simulink model "sim_controller_from_ground"  (R2024b)
settings: Solver=ode1be  StartTime=t_0  StopTime=100  FixedStep=dt  RelTol=1e-8
undefined symbols (not defined in the file or in its folder): controller_rate
libraries: simulink x1
settings Model: Creator=yevge  LastModifiedBy=Aiden Gaydos
settings DebuggingCC: AlgebraicLoopMsg=error  CheckMatrixSingularityMsg=error

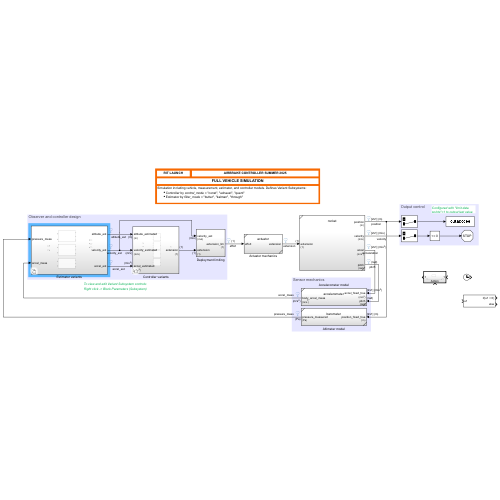
[thumbnail: Simulink's stored preview of the top-level diagram]
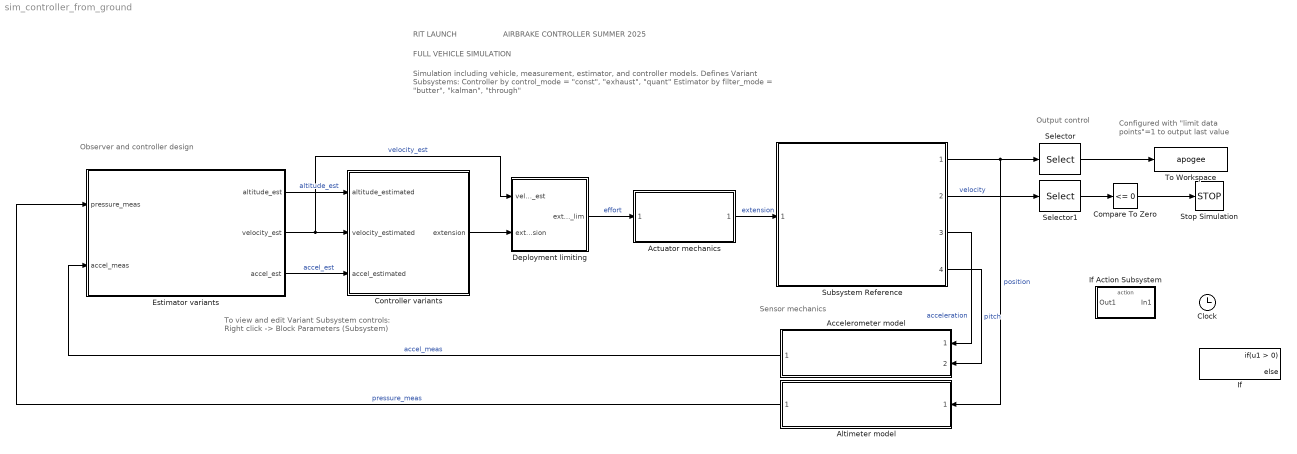
== system sim_controller_from_ground ==
  note: Output control
  note: Configured with "limit data points"=1 to output last value
  note: Sensor mechanics
  note: Observer and controller design
  note: AIRBRAKE CONTROLLER SUMMER 2025
  note: Simulation including vehicle, measurement, estimator, and controller models. Defines Variant Subsystems:
      | Controller by control_mode = "const", "exhaust", "quant"
      | Estimator by filter_mode = "butter", "kalman", "through"
  note: RIT LAUNCH
  note: FULL VEHICLE SIMULATION
  note: To view and edit Variant Subsystem controls:
      | Right click -> Block Parameters (Subsystem)
  Accelerometer model : Subsystem  ReferencedSubsystem=accelerometer
  Actuator mechanics : Subsystem  ReferencedSubsystem=actuator
  Altimeter model : Subsystem  ReferencedSubsystem=barometer
  Clock : Clock
  Compare To Zero : simulink/Logic and Bit Operations/Compare To Zero  relop=<=  OutDataTypeStr=boolean
  Controller variants : Subsystem  Variant=on  VariantControl=Subsystem  AllowZeroVariantControls=on
  Deployment limiting : Subsystem
  Estimator variants : Subsystem  Variant=on  VariantControl=Signal processing  AllowZeroVariantControls=on
  If : If
  If Action Subsystem : Subsystem  TreatAsAtomicUnit=on
  Selector : Selector  InputPortWidth=2  IndexOptions=Index vector (dialog)  Indices=2  OutputSizes=1
  Selector1 : Selector  InputPortWidth=2  IndexOptions=Index vector (dialog)  Indices=2  OutputSizes=1
  Stop Simulation : Stop
  Subsystem Reference : Subsystem  ReferencedSubsystem=rocket
  To Workspace : ToWorkspace  VariableName=apogee  SampleTime=-1
      settings: MaxDataPoints=1
  wires:
  Subsystem Reference/3 -> Accelerometer model/1  "acceleration"
  Subsystem Reference/4 -> Accelerometer model/2  "pitch"
  Subsystem Reference/1 -> Selector/1, Altimeter model/1  "position"
  Selector1/1 -> Compare To Zero/1
  Compare To Zero/1 -> Stop Simulation/1
  Selector/1 -> To Workspace/1
  Subsystem Reference/2 -> Selector1/1  "velocity"
  Controller variants/1(extension) -> Deployment limiting/2(extension)
  Deployment limiting/1(extension_lim) -> Actuator mechanics/1  "effort"
  Actuator mechanics/1 -> Subsystem Reference/1  "extension"
  Accelerometer model/1 -> Estimator variants/2(accel_meas)  "accel_meas"
  Estimator variants/1(altitude_est) -> Controller variants/1(altitude_estimated)  "altitude_est"
  Estimator variants/2(velocity_est) -> Controller variants/2(velocity_estimated), Deployment limiting/1(velocity_est)  "velocity_est"
  Estimator variants/3(accel_est) -> Controller variants/3(accel_estimated)  "accel_est"
  Altimeter model/1 -> Estimator variants/1(pressure_meas)  "pressure_meas"

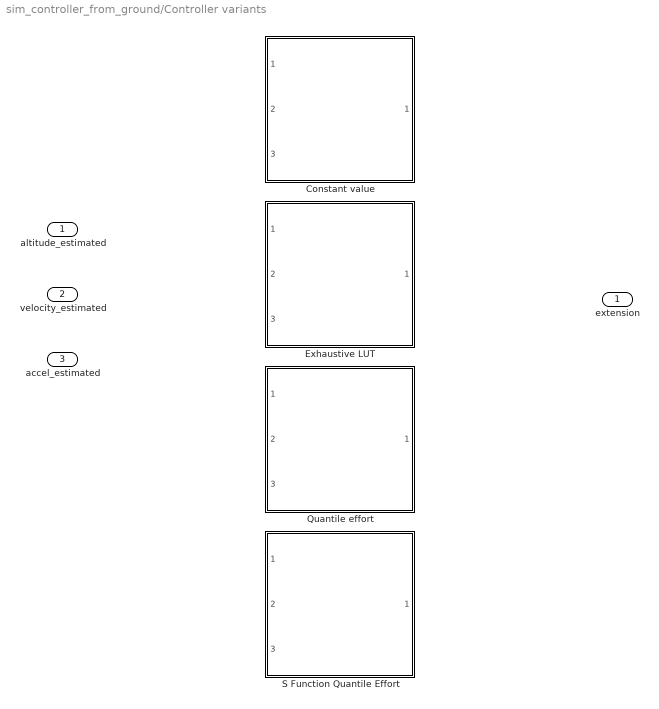
== system sim_controller_from_ground/Controller variants ==
  altitude_estimated : Inport  Unit=m  PortDimensions=1  SampleTime=1/controller_rate
  velocity_estimated : Inport  Port=2  Unit=m/s  PortDimensions=1  SampleTime=1/controller_rate
  accel_estimated : Inport  Port=3  Unit=m/s^2  PortDimensions=1  SampleTime=1/controller_rate
  Constant value : Subsystem  VariantControl="control_mode == \"const\""  ReferencedSubsystem=const_controller
  Exhaustive LUT : Subsystem  VariantControl="control_mode == \"exhaust\""  ReferencedSubsystem=exhaust_lut_controller
  Quantile effort : Subsystem  VariantControl="control_mode == \"quant\""  ReferencedSubsystem=quantile_effort_controller
  S Function Quantile Effort : Subsystem  VariantControl="control_mode == \"s\""  ReferencedSubsystem=s_function_quantile_effort_controller
  extension : Outport  OutMin=0  OutMax=1  Unit=1  PortDimensions=1  SampleTime=1/controller_rate

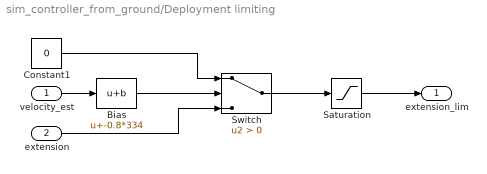
== system sim_controller_from_ground/Deployment limiting ==
  velocity_est : Inport  Unit=m/s  PortDimensions=1
  extension : Inport  Port=2  OutMin=0  OutMax=1  Unit=1  PortDimensions=1
  Bias : Bias  Bias=-0.8*334  SaturateOnIntegerOverflow=off
  Constant1 : Constant  Value=0
  Saturation : Saturate  UpperLimit=1  LowerLimit=0
  Switch : Switch  Criteria=u2 > Threshold  SaturateOnIntegerOverflow=off  InputSameDT=off
  extension_lim : Outport  OutMin=0  OutMax=1  Unit=1  PortDimensions=1
  wires:
  Constant1/1 -> Switch/1
  extension/1 -> Switch/3
  velocity_est/1 -> Bias/1
  Bias/1 -> Switch/2
  Saturation/1 -> extension_lim/1
  Switch/1 -> Saturation/1

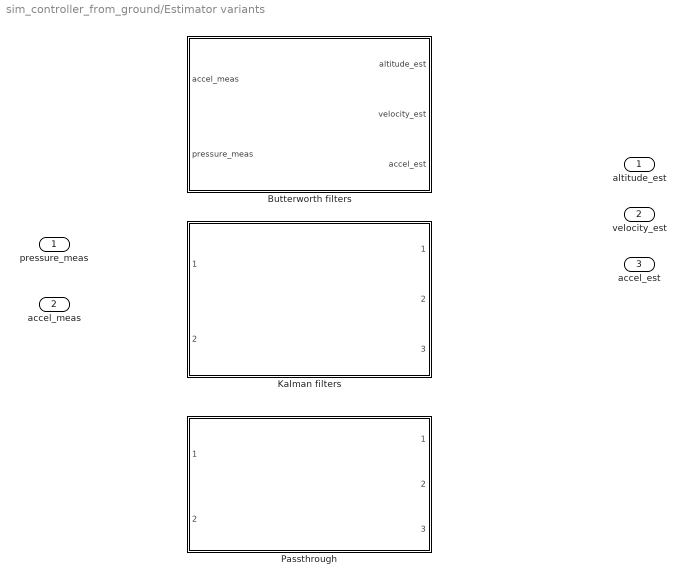
== system sim_controller_from_ground/Estimator variants ==
  pressure_meas : Inport  PortDimensions=1
  accel_meas : Inport  Port=2  PortDimensions=1
  Butterworth filters : Subsystem  VariantControl="filter_mode == \"butter\""
  Kalman filters : Subsystem  VariantControl="filter_mode == \"kalman\""  ReferencedSubsystem=kalman_filter
  Passthrough : Subsystem  VariantControl="filter_mode == \"through\""  ReferencedSubsystem=no_filter
  altitude_est : Outport  PortDimensions=1
  velocity_est : Outport  Port=2  PortDimensions=1
  accel_est : Outport  Port=3  PortDimensions=1

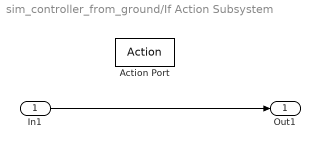
== system sim_controller_from_ground/If Action Subsystem ==
  In1 : Inport
  Action Port : ActionPort
  Out1 : Outport
  wires:
  In1/1 -> Out1/1

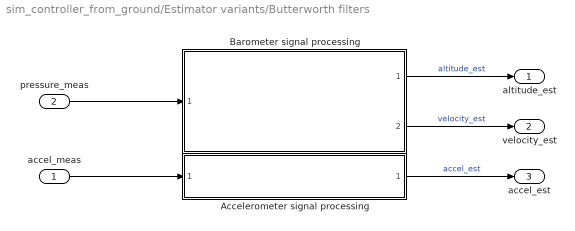
== system sim_controller_from_ground/Estimator variants/Butterworth filters ==
  accel_meas : Inport
  pressure_meas : Inport  Port=2
  Accelerometer signal processing : Subsystem  ReferencedSubsystem=accel_filter
  Barometer signal processing : Subsystem  ReferencedSubsystem=baro_filters
  altitude_est : Outport
  velocity_est : Outport  Port=2
  accel_est : Outport  Port=3
  wires:
  Barometer signal processing/2 -> velocity_est/1  "velocity_est"
  Barometer signal processing/1 -> altitude_est/1  "altitude_est"
  pressure_meas/1 -> Barometer signal processing/1
  accel_meas/1 -> Accelerometer signal processing/1
  Accelerometer signal processing/1 -> accel_est/1  "accel_est"
